simulink model "DiffEq_Solver_Model"  (R2020a)
settings: Solver=VariableStepAuto  StartTime=0.0  StopTime=10.0  RelTol=1e-3
values from neighbouring files (symbols this model uses):
  A = 3    [DiffEq_Solver_mScript.m]
  F = 2    [DiffEq_Solver_mScript.m]
  Ti = 0.5    [DiffEq_Solver_mScript.m]
settings Model: Creator=alexd  LastModifiedBy=alexd

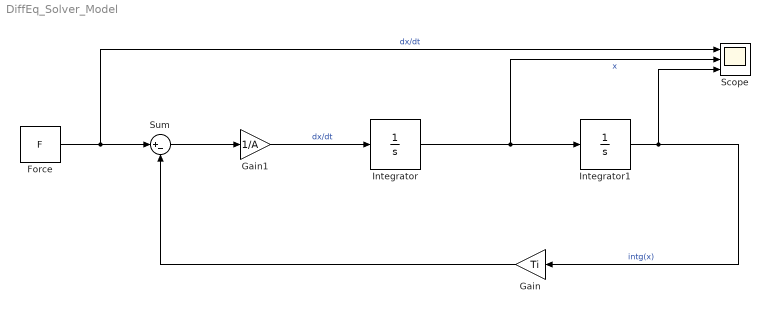
== system DiffEq_Solver_Model ==
  Force : Constant  Value=F
  Gain : Gain  Gain=Ti
  Gain1 : Gain  Gain=1/A
  Integrator : Integrator
  Integrator1 : Integrator
  Scope : Scope  NumInputPorts=3
  Sum : Sum  Inputs=|+-
  wires:
  Gain1/1 -> Integrator/1  "dx/dt"
  Integrator/1 -> Scope/2, Integrator1/1  "x"
  Integrator1/1 -> Scope/3, Gain/1  "intg(x)"
  Force/1 -> Scope/1, Sum/1  "dx/dt"
  Gain/1 -> Sum/2
  Sum/1 -> Gain1/1
